simulink library "Lib_Vol_Valve_TMATS"  (R2015a)
settings: Solver=ode45  StartTime=0.0  StopTime=10.0  RelTol=1e-3
undefined symbols (not defined in the file): Fluid
libraries: Lib_Vol_PropLookup_TMATS x3, simulink x1
Description:
  | Thomas Modules
settings Model: CovSFcnEnable=off  Creator=jwchapm2  LastModifiedBy=jwchapm2
settings OptimizationCC: ExpressionDepthLimit=2147483647
settings DebuggingCC: UnderspecifiedInitializationDetection=Classic  MergeDetectMultiDrivingBlocksExec=none  SolverPrmCheckMsg=warning  StateNameClashWarn=warning

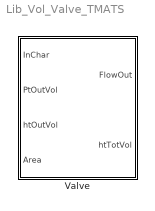
== system Lib_Vol_Valve_TMATS ==
  Valve : Subsystem  mask(T-MATS: Valve Library Block){Cd_M=0.6, htVec_M=Fluid.Vec.ht, PtVec_M=Fluid.Vec.Pt, TtArray_M=Fluid.Array.Tt, rhoArray_M=Fluid.Array.rho}
      mask prompts: Cd_M "Cd_M - Discharge coefficient (unitless)"; htVec_M "htVec_M - Temperature Vector"; PtVec_M "PtVec_M - Pressure Vector"; TtArray_M "TtArray_M - Temperature Array"; rhoArray_M "rhoArray_M - density"
      mask help: This block simulates the performance of a valve using basic fluid dynamic equations and properties.
      mask Help: web(which('Vol_TMATS_Valve.html'),'-helpbrowser')

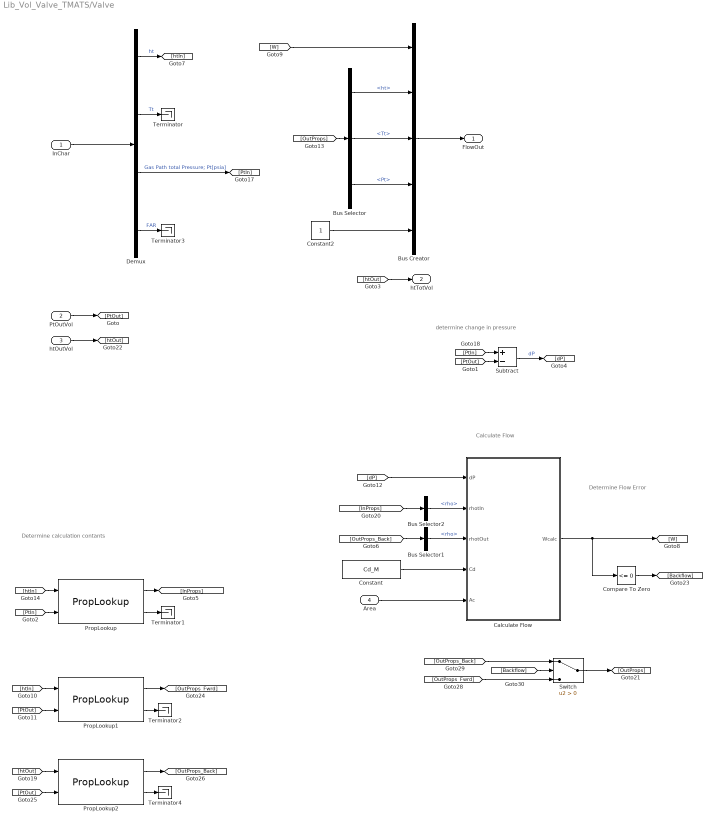
== system Lib_Vol_Valve_TMATS/Valve ==
  note: determine change in pressure
  note: Determine Flow Error
  note: Determine calculation contants
  note: Calculate Flow
  InChar : Inport
  PtOutVol : Inport  Port=2
  htOutVol : Inport  Port=3
  Area : Inport  Port=4
  Bus Selector : BusSelector  OutputSignals=ht,Tt,Pt
  Bus Selector1 : BusSelector  OutputSignals=rho
  Bus Selector2 : BusSelector  OutputSignals=rho
  Bus Creator : BusCreator  Inputs=5
  Calculate Flow : MATLAB Function  TreatAsAtomicUnit=on
  Compare To Zero : simulink/Logic and Bit Operations/Compare To Zero  relop=<=  OutDataTypeStr=boolean
  Constant : Constant  Value=Cd_M
  Constant2 : Constant
  Demux : Demux
  PropLookup : Lib_Vol_PropLookup_TMATS/PropLookup  case_M='ht'  propg_M=0  htg_M=0  htVec_M=htVec_M  PtVec_M=PtVec_M  TtVec_M=[-1000 1000]  sVec_M=[-1000 1000]  htArray_M=ones(2,length(PtVec_M))'  rhoArray_M=rhoArray_M  uArray_M=ones(length(htVec_M), length(PtVec_M))'  sArray_M=ones(length(htVec_M), length(PtVec_M))'  muArray_M=ones(length(htVec_M), length(PtVec_M))'  ThArray_M=TtArray_M  CvArray_M=ones(length(htVec_M), length(PtVec_M))'  CpArray_M=ones(length(htVec_M), length(PtVec_M))'  kArray_M=ones(length(htVec_M), length(PtVec_M))'  TsArray_M=ones(2, length(PtVec_M))'  hsArray_M=ones(2, length(PtVec_M))'  Rval_M=0.000
  PropLookup1 : Lib_Vol_PropLookup_TMATS/PropLookup  case_M='ht'  propg_M=0  htg_M=0  htVec_M=htVec_M  PtVec_M=PtVec_M  TtVec_M=[-1000 1000]  sVec_M=[-1000 1000]  htArray_M=ones(2,length(PtVec_M))'  rhoArray_M=rhoArray_M  uArray_M=ones(length(htVec_M), length(PtVec_M))'  sArray_M=ones(length(htVec_M), length(PtVec_M))'  muArray_M=ones(length(htVec_M), length(PtVec_M))'  ThArray_M=TtArray_M  CvArray_M=ones(length(htVec_M), length(PtVec_M))'  CpArray_M=ones(length(htVec_M), length(PtVec_M))'  kArray_M=ones(length(htVec_M), length(PtVec_M))'  TsArray_M=ones(2, length(PtVec_M))'  hsArray_M=ones(2, length(PtVec_M))'  Rval_M=0.000
  PropLookup2 : Lib_Vol_PropLookup_TMATS/PropLookup  case_M='ht'  propg_M=0  htg_M=0  htVec_M=htVec_M  PtVec_M=PtVec_M  TtVec_M=[-1000 1000]  sVec_M=[-1000 1000]  htArray_M=ones(2,length(PtVec_M))'  rhoArray_M=rhoArray_M  uArray_M=ones(length(htVec_M), length(PtVec_M))'  sArray_M=ones(length(htVec_M), length(PtVec_M))'  muArray_M=ones(length(htVec_M), length(PtVec_M))'  ThArray_M=TtArray_M  CvArray_M=ones(length(htVec_M), length(PtVec_M))'  CpArray_M=ones(length(htVec_M), length(PtVec_M))'  kArray_M=ones(length(htVec_M), length(PtVec_M))'  TsArray_M=ones(2, length(PtVec_M))'  hsArray_M=ones(2, length(PtVec_M))'  Rval_M=0.000
  Subtract : Sum  Inputs=+-
  Switch : Switch  Criteria=u2 > Threshold
  Terminator{,1..4} (5 alike) : Terminator
  FlowOut : Outport  PortDimensions=5
  htTotVol : Outport  Port=2  PortDimensions=1
  wires:
  Area/1 -> Calculate Flow/5(Ac)
  Constant2/1 -> Bus Creator/5
  Demux/4 -> Terminator3/1  "FAR"
  [htOut] -> htTotVol/1
  Bus Selector/2 -> Bus Creator/3  "<Tt>"
  [htOut] -> PropLookup2/1
  [PtOut] -> PropLookup2/2
  PropLookup2/2 -> Terminator4/1
  PropLookup2/1 -> [OutProps_Back]
  htOutVol/1 -> [htOut]
  Demux/2 -> Terminator/1  "Tt"
  [Backflow] -> Switch/2
  [OutProps_Fwrd] -> Switch/3
  [OutProps_Back] -> Switch/1
  Switch/1 -> [OutProps]
  Compare To Zero/1 -> [Backflow]
  [W] -> Bus Creator/1
  Bus Selector2/1 -> Calculate Flow/2(rhotIn)  "<rho>"
  [InProps] -> Bus Selector2/1
  [htIn] -> PropLookup1/1
  [PtOut] -> PropLookup1/2
  PropLookup1/2 -> Terminator2/1
  PropLookup1/1 -> [OutProps_Fwrd]
  [PtIn] -> Subtract/1
  Constant/1 -> Calculate Flow/4(Cd)
  [htIn] -> PropLookup/1
  [OutProps] -> Bus Selector/1
  [dP] -> Calculate Flow/1(dP)
  Bus Selector1/1 -> Calculate Flow/3(rhotOut)  "<rho>"
  Calculate Flow/1(Wcalc) -> [W], Compare To Zero/1
  [OutProps_Back] -> Bus Selector1/1
  Bus Selector/3 -> Bus Creator/4  "<Pt>"
  [PtIn] -> PropLookup/2
  [PtOut] -> Subtract/2
  PtOutVol/1 -> [PtOut]
  Bus Selector/1 -> Bus Creator/2  "<ht>"
  PropLookup/2 -> Terminator1/1
  PropLookup/1 -> [InProps]
  Demux/1 -> [htIn]  "ht"
  Subtract/1 -> [dP]  "dP"
  Demux/3 -> [PtIn]  "Gas Path total Pressure; Pt[psia]"
  Bus Creator/1 -> FlowOut/1
  InChar/1 -> Demux/1

== matlab function Lib_Vol_Valve_TMATS/Valve/Calculate Flow ==
  data: dP input; Wcalc output; rhotIn input; rhotOut input; Cd input; Ac input
function Wcalc = fcn(dP,rhotIn,rhotOut,Cd,Ac)
%Calculate flow
g = 32.174049;
if dP > 0
    Wcalc = Cd*Ac*sqrt(2*g*dP*(rhotIn/12/12/12));
else
    Wcalc = -Cd*Ac*sqrt(2*g*-dP*(rhotOut/12/12/12));
end
